simulink model "ON_toggling_led"  (R2022b)
settings: Solver=FixedStepDiscrete  StartTime=0.0  StopTime=10.0  FixedStep=0.1  RelTol=1e-3  EnableMultiTasking=on
settings Model: DVExtractedSubsystem=ON.toggling_led  Creator=alewi  LastModifiedBy=alewi
settings SolverCC: AlgebraicLoopSolver=TrustRegion  AutoInsertRateTranBlk=on
settings DataIOCC: LimitDataPoints=on
settings OptimizationCC: LifeSpan=inf
settings DebuggingCC: UnconnectedInputMsg=warning  UnconnectedOutputMsg=warning  UnconnectedLineMsg=warning  FrameProcessingCompatibilityMsg=none  AllowSymbolicDim=off  SFUnexpectedBacktrackingDiag=warning  SFNoUnconditionalDefaultTransitionDiag=warning  SFExecutionAtInitializationDiag=none  ArithmeticOperatorsInVariantConditions=warning
settings ModelReferenceCC: EnableRefExpFcnMdlSchedulingChecks=on
settings SFSimCC: SimUseLocalCustomCode=off  CustomCodeUndefinedFunction=UseInterfaceOnly
settings RTWCC: TLCOptions=-aAlwaysIncludeCustomSrc=1  RTWUseLocalCustomCode=off  DLArmComputeVersion=19.05
settings CodeAppCC: StateflowObjectComments=on
settings GRTTargetCC: TargetLangStandard=C89/C90 (ANSI)
settings ConfigComp: CovMetricSettings=dw  CovSaveCumulativeToWorkspaceVar=on  CovSaveSingleToWorkspaceVar=on  CovExternalEMLEnable=off  CovSFcnEnable=off  DVTestSuiteOptimization=Auto  DVDetectOutOfBounds=on  DVModelReferenceHarness=on  DVHarnessSource=Signal Editor

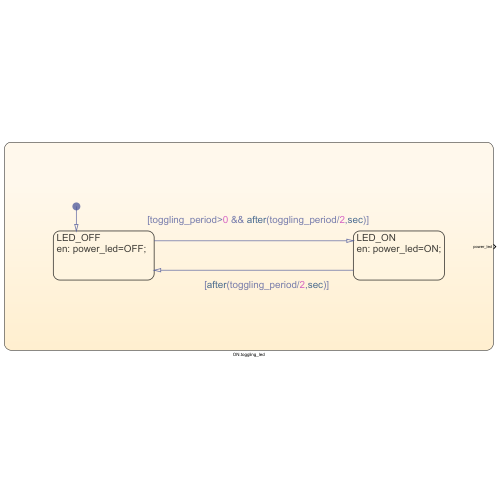
[thumbnail: Simulink's stored preview of the top-level diagram]
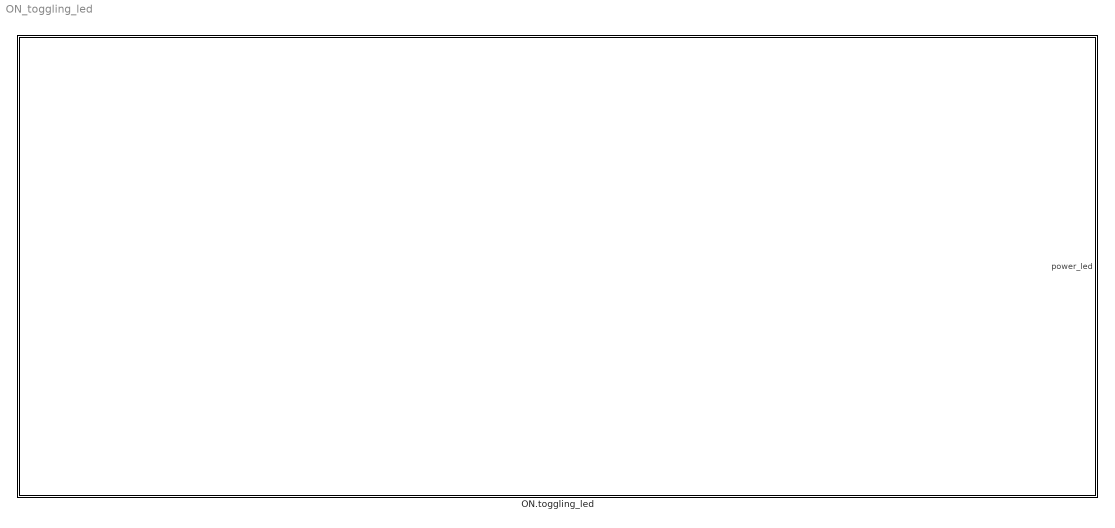
== system ON_toggling_led ==
  ON.toggling_led : Stateflow chart  Priority=1  TreatAsAtomicUnit=on

== stateflow chart ON_toggling_led/ON.toggling_led ==
  state LED_OFF
    en: power_led=OFF;
  state LED_ON
    en: power_led=ON;
  (default) -> LED_OFF
  LED_OFF -> LED_ON : [toggling_period>0 && after(toggling_period/2,sec)]
  LED_ON -> LED_OFF : [after(toggling_period/2,sec)]
  data: toggling_period data_store_memory size=1; power_led output boolean size=1; OFF constant boolean size=1 =0; ON constant boolean size=1 =1
